simulink model "sampleModel1"  (R2021a)
settings: Solver=VariableStepAuto  StartTime=0.0  StopTime=50  RelTol=1e-3
undefined symbols (not defined in the file): DiscIntNeverNeededParam, magnitude, Newton, Raphson
libraries: simulink x92, pid_lib x10
(part 1 of 5)
settings Model: SimulationMode=accelerator  Creator=user  LastModifiedBy=O1

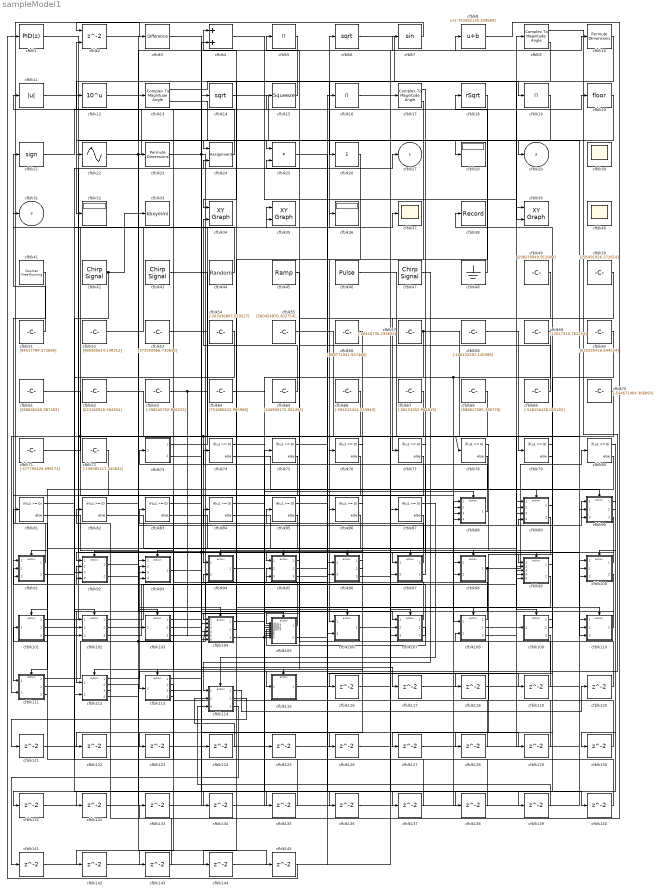
== system sampleModel1 ==
  cfblk1 : pid_lib/PID Controller  Controller=PID  Form=Parallel  TimeDomain=Discrete-time  UseExternalTs=off  SampleTime=1  IntegratorMethod=Forward Euler  FilterMethod=Forward Euler  ControllerParametersSource=internal  P=1  I=1  D=0  UseFilter=on  N=100  TunerSelectOption=Transfer Function Based (PID Tuner App)  InitialConditionSource=internal  InitialConditionForIntegrator=0  InitialConditionForFilter=0  DifferentiatorICPrevScaledInput=0  ExternalReset=none  TrackingMode=off  Kt=1  LimitOutput=off  SatLimitsSource=internal  UpperSaturationLimit=inf  LowerSaturationLimit=-inf  LinearizeAsGain=off  AntiWindupMode=none  Kb=1  POutMin=[]  POutMax=[]  IOutMin=[]  IOutMax=[]  DOutMin=[]  DOutMax=[]  NOutMin=[]  NOutMax=[]  SumOutMin=[]  SumOutMax=[]  SaturationOutMin=[]  SaturationOutMax=[]  PParamMin=[]  PParamMax=[]  IParamMin=[]  IParamMax=[]  DParamMin=[]  DParamMax=[]  NParamMin=[]  NParamMax=[]  KbParamMin=[]  KbParamMax=[]  KtParamMin=[]  KtParamMax=[]  KbOutMin=[]  KbOutMax=[]  KtOutMin=[]  KtOutMax=[]  IntegratorOutMin=[]  IntegratorOutMax=[]  FilterOutMin=[]  FilterOutMax=[]  SumI1OutMin=[]  SumI1OutMax=[]  SumI2OutMin=[]  SumI2OutMax=[]  SumI3OutMin=[]  SumI3OutMax=[]  SumI4OutMin=[]  SumI4OutMax=[]  SumDOutMin=[]  SumDOutMax=[]  DifferentiatorOutMin=[]  DifferentiatorOutMax=[]  FilterDiffOutCoefMin=[]  FilterDiffOutCoefMax=[]  ReciprocalOutMin=[]  ReciprocalOutMax=[]  SumDenOutMin=[]  SumDenOutMax=[]  SumNumOutMin=[]  SumNumOutMax=[]  DivideOutMin=[]  DivideOutMax=[]  UdiffTsProdOutMin=[]  UdiffTsProdOutMax=[]  NTsProdOutMin=[]  NTsProdOutMax=[]  UintegralTsProdOutMin=[]  UintegralTsProdOutMax=[]  UngainTsProdOutMin=[]  UngainTsProdOutMax=[]  IntegratorContinuousStateAttributes=''  IntegratorStateMustResolveToSignalObject=off  IntegratorRTWStateStorageClass=Auto  FilterContinuousStateAttributes=''  FilterStateMustResolveToSignalObject=off  FilterRTWStateStorageClass=Auto  ParallelPVariant=InternalParameters  IdealPVariant=Disabled  IVariant=InternalParameters  DVariant=InternalParameters  IntegratorVariant=Discrete  SatVariant=Disabled  AWVariant=Passthrough  PCopyVariant=Disabled  TRVariant=Disabled  FdbkBlocksVariant=Forward  IdealPFdbkVariant=Disabled  SatFdbkVariant=Disabled  DerivativeFilterVariant=ForwardEulerFilter  NVariant=InternalParameters  NCopyVariant=Disabled  FilterICVariant=InternalICsFilter  IntegratorICVariant=InternalICs  ExternalResetVariant=Disabled  TRSumVariant=Passthrough  SumFdbkVariant=Disabled  SumVariant=Sum_PID  TsampFilterVariant=InternalTs  TsampNgainVariant=Passthrough  TsampIntegralVariant=Passthrough  ExternalSaturationOutDataTypeStr=Inherit: Same as second input
  cfblk10 : PermuteDimensions
  cfblk100 : Subsystem  TreatAsAtomicUnit=on
  cfblk101 : Subsystem  TreatAsAtomicUnit=on
  cfblk102 : Subsystem  TreatAsAtomicUnit=on
  cfblk103 : Subsystem  TreatAsAtomicUnit=on
  cfblk104 : Subsystem  TreatAsAtomicUnit=on
  cfblk105 : Subsystem  TreatAsAtomicUnit=on
  cfblk106 : Subsystem  TreatAsAtomicUnit=on
  cfblk107 : Subsystem  TreatAsAtomicUnit=on
  cfblk108 : Subsystem  TreatAsAtomicUnit=on
  cfblk109 : Subsystem  TreatAsAtomicUnit=on
  cfblk11 : Abs
  cfblk110 : Subsystem  TreatAsAtomicUnit=on
  cfblk111 : Subsystem  TreatAsAtomicUnit=on
  cfblk112 : Subsystem  TreatAsAtomicUnit=on
  cfblk113 : Subsystem  TreatAsAtomicUnit=on
  cfblk114 : Subsystem  TreatAsAtomicUnit=on
  cfblk115 : Subsystem  TreatAsAtomicUnit=on
  cfblk{116..145} (30 alike) : Delay  SampleTime=1
  cfblk12 : Math  Operator=10^u  SaturateOnIntegerOverflow=on
  cfblk13 : ComplexToMagnitudeAngle
  cfblk14 : Sqrt  SaturateOnIntegerOverflow=on
  cfblk15 : Squeeze
  cfblk16 : Product  Inputs=*
  cfblk17 : ComplexToMagnitudeAngle
  cfblk18 : Sqrt  Operator=rSqrt  AlgorithmType=Newton-Raphson  SaturateOnIntegerOverflow=on
  cfblk19 : Product  Inputs=*
  cfblk2 : Delay  ShowEnablePort=on  SampleTime=1
      settings: InputPortMap=u0,e6
  cfblk20 : Rounding
  cfblk21 : Signum
  cfblk22 : Sin  TimeSource=Use external signal  SampleTime=0
  cfblk23 : PermuteDimensions
  cfblk24 : Assignment  DiagnosticForDimensions=Warning  IndexOptions=Index vector (dialog)  Indices=1  OutputSizes=1
  cfblk25 : DotProduct  InputSameDT=on  OutDataTypeStr=Inherit: Inherit via internal rule
  cfblk26 : Sum  Inputs=+
  cfblk28 : Display
  cfblk3 : simulink/Discrete/Difference  ICPrevInput=0.0  OutMin=[]  OutMax=[]  OutDataTypeStr=Inherit: Inherit via back propagation  OutDataType=fixdt(1, 16)  OutScaling=2^-10  DoSatur=off
  cfblk30 : Scope
      settings: Floating=on
  cfblk32 : Display
  cfblk33 : ToWorkspace  VariableName=kbxymmi  SaveFormat=Timeseries  SampleTime=-1
  cfblk34 : simulink/Sinks/XY Graph  xmin=-1  xmax=1  ymin=-1  ymax=1  st=-1
  cfblk35 : simulink/Sinks/XY Graph  xmin=-1  xmax=1  ymin=-1  ymax=1  st=-1
  cfblk36 : Display
  cfblk37 : Scope
  cfblk38 : Record  FileSettingsInternal="{\"entries\":[{\"content\":{\"excelSettings\":{\"content\":{},\"type\":\"Streamout.ExcelSettings\"}},\"type\":\"Streamout.FileSettingStorage\",\"uuid\":\"176fac1a-9541-496c-8a8b-0fabc606d681\"}],\"packageUris\":[\"http://schema.mathworks.com/mf0/streamout_blocks/R2020a\"],\"version\":\"1.0\"}"  SignalsInternal="{\"entries\":[{\"content\":{\"signals\":[{\"content\":{\"blockPath\":[\"sampleModel1/cfblk38\"],\"channel\":[],\"dimensions\":[1],\"domain\":\"samplemodel1/cfblk38\",\"lineColor\":\"#ff6929\",\"plots\":[1],\"port\":1,\"sid\":[],\"signalID\":15,\"signalName\":\"cfblk109:2\"},\"type\":\"RecordBlkView.Signal\",\"uuid\":\"c7513c56-5db2-4e4b-af3b-43bbc007c584\"}]},\"type\":\"RecordBlkView.InputSignals\",\"uuid\":\"33f00b58-3736-4c4e-bce4-d943bd5669e6\"}],\"packageUris\":[\"http://schema.mathworks.com/mf0/streamout_blocks/R2020a\"],\"version\":\"1.0\"}"  VisualizationBindings="{\"sparklinesplugin\":{\"info\":[{\"bindingParametersList\":[],\"subplotID\":1}]}}"
  cfblk39 : simulink/Sinks/XY Graph  xmin=-1  xmax=1  ymin=-1  ymax=1  st=-1
  cfblk4 : Sum
  cfblk40 : Scope
      settings: Floating=on
  cfblk41 : simulink/Sources/Counter Free-Running  NumBits=[54.000000]  tsamp=-1
  cfblk42 : simulink/Sources/Chirp Signal  f1=[-261506437.759570]  T=[-777594489.412425]  f2=[560504136.642276]
  cfblk43 : simulink/Sources/Chirp Signal  f1=[-220522326.077493]  T=[-516617428.172335]  f2=[-192175708.823771]
  cfblk44 : RandomNumber  Mean=[-80709.094966]  Variance=[13197.329261]  Seed=[942050590.000000]  SampleTime=0.1
  cfblk45 : simulink/Sources/Ramp  slope=[9122.690805]  start=[29.185221]  InitialOutput=[-880440.914106]
  cfblk46 : DiscretePulseGenerator  PulseType=Time based  Amplitude=[-530440173.255187]  Period=[35315857.769049]  PulseWidth=5  PhaseDelay=[8.000000]
  cfblk47 : simulink/Sources/Chirp Signal  f1=[-969193124.696890]  T=[-913952396.684384]  f2=[-662019941.074591]
  cfblk48 : Ground
  cfblk49 : Constant  Value=[298230949.912904]  SampleTime=1
  cfblk5 : Product  Inputs=*
  cfblk50 : Constant  Value=[295491926.272614]  SampleTime=1
  cfblk51 : Constant  Value=[94017784.572690]  SampleTime=1
  cfblk52 : Constant  Value=[489385614.148312]  SampleTime=1
  cfblk53 : Constant  Value=[373550866.730630]  SampleTime=1
  cfblk54 : Constant  Value=[-263030807.019327]  SampleTime=1
  cfblk55 : Constant  Value=[560454870.302754]  SampleTime=1
  cfblk56 : Constant  Value=[858771941.937460]  SampleTime=1
  cfblk57 : Constant  Value=[-26416735.193655]  SampleTime=1
  cfblk58 : Constant  Value=[-106432501.140388]  SampleTime=1
  cfblk59 : Constant  Value=[17017310.762254]  SampleTime=1
  cfblk6 : Sqrt  SaturateOnIntegerOverflow=on
  cfblk60 : Constant  Value=[635255416.644524]  SampleTime=1
  cfblk61 : Constant  Value=[288636260.387383]  SampleTime=1
  cfblk62 : Constant  Value=[623160916.564954]  SampleTime=1
  cfblk63 : Constant  Value=[-298545792.846233]  SampleTime=1
  cfblk64 : Constant  Value=[751885622.985968]  SampleTime=1
  cfblk65 : Constant  Value=[244950172.002455]  SampleTime=1
  cfblk66 : Constant  Value=[-584515414.533943]  SampleTime=1
  cfblk67 : Constant  Value=[-58153302.964819]  SampleTime=1
  cfblk68 : Constant  Value=[688617585.390778]  SampleTime=1
  cfblk69 : Constant  Value=[-548156438.055202]  SampleTime=1
  cfblk7 : Trigonometry
  cfblk70 : Constant  Value=[-544671404.366893]  SampleTime=1
  cfblk71 : Constant  Value=[-377795426.699174]  SampleTime=1
  cfblk72 : Constant  Value=[-139585217.340832]  SampleTime=1
  cfblk73 : Subsystem
  cfblk{74..87} (14 alike) : If  IfExpression=u1 >= 0  SampleTime=1
  cfblk8 : Bias  Bias=[-753362130.329669]
  cfblk88 : Subsystem  TreatAsAtomicUnit=on
  cfblk89 : Subsystem  TreatAsAtomicUnit=on
  cfblk9 : ComplexToMagnitudeAngle
  cfblk90 : Subsystem  TreatAsAtomicUnit=on
  cfblk91 : Subsystem  TreatAsAtomicUnit=on
  cfblk92 : Subsystem  TreatAsAtomicUnit=on
  cfblk93 : Subsystem  TreatAsAtomicUnit=on
  cfblk94 : Subsystem  TreatAsAtomicUnit=on
  cfblk95 : Subsystem  TreatAsAtomicUnit=on
  cfblk96 : Subsystem  TreatAsAtomicUnit=on
  cfblk97 : Subsystem  TreatAsAtomicUnit=on
  cfblk98 : Subsystem  TreatAsAtomicUnit=on
  cfblk99 : Subsystem  TreatAsAtomicUnit=on
  cfblk27 : Outport
  cfblk29 : Outport  Port=2
  cfblk31 : Outport  Port=3
  wires:
  cfblk42/1 -> cfblk33/1, cfblk102/3(cfblk10)
  cfblk98/1(cfblk2) -> cfblk80/1, cfblk104/6(cfblk15)
  cfblk1/1 -> cfblk100/2(cfblk8)
  cfblk91/1(cfblk2) -> cfblk3/1
  cfblk61/1 -> cfblk78/1, cfblk99/3(cfblk12)
  cfblk13/1 -> cfblk19/1
  cfblk9/1 -> cfblk115/1(cfblk1)
  cfblk73/1(cfblk2) -> cfblk6/1
  cfblk14/1 -> cfblk28/1
  cfblk52/1 -> cfblk37/1
  cfblk97/1(cfblk2) -> cfblk85/1
  cfblk13/2 -> cfblk110/1(cfblk1)
  cfblk51/1 -> cfblk21/1
  cfblk47/1 -> cfblk114/1(cfblk1)
  cfblk23/1 -> cfblk99/4(cfblk13), cfblk105/7(cfblk12), cfblk107/1(cfblk1)
  cfblk115/1(cfblk2) -> cfblk17/1
  cfblk72/1 -> cfblk111/1(cfblk1)
  cfblk49/1 -> cfblk77/1
  cfblk100/1(cfblk2) -> cfblk97/1(cfblk1)
  cfblk7/1 -> cfblk2/1
  cfblk101/1(cfblk2) -> cfblk27/1
  cfblk71/1 -> cfblk13/1
  cfblk10/1 -> cfblk26/1
  cfblk68/1 -> cfblk106/1(cfblk1)
  cfblk19/1 -> cfblk25/1
  cfblk9/2 -> cfblk32/1
  cfblk41/1 -> cfblk91/1(cfblk1)
  cfblk46/1 -> cfblk98/1(cfblk1)
  cfblk6/1 -> cfblk39/1
  cfblk24/1 -> cfblk2/2
  cfblk11/1 -> cfblk24/1
  cfblk5/1 -> cfblk34/1
  cfblk16/1 -> cfblk10/1
  cfblk55/1 -> cfblk108/1(cfblk1)
  cfblk59/1 -> cfblk88/2(cfblk8), cfblk105/6(cfblk11)
  cfblk100/2(cfblk10) -> cfblk112/1(cfblk1)
  cfblk62/1 -> cfblk94/1(cfblk1), cfblk99/5(cfblk14)
  cfblk20/1 -> cfblk22/1
  cfblk111/1(cfblk2) -> cfblk16/1
  cfblk108/1(cfblk2) -> cfblk4/1
  cfblk105/1(cfblk2) -> cfblk84/1
  cfblk58/1 -> cfblk79/1
  cfblk60/1 -> cfblk99/1(cfblk1)
  cfblk45/1 -> cfblk105/1(cfblk1)
  cfblk102/1(cfblk2) -> cfblk14/1
  cfblk70/1 -> cfblk107/3(cfblk14)
  cfblk108/2(cfblk11) -> cfblk89/2(cfblk12)
  cfblk73/2(cfblk16) -> cfblk36/1
  cfblk88/1(cfblk2) -> cfblk25/2
  cfblk12/1 -> cfblk7/1
  cfblk95/1(cfblk2) -> cfblk94/2(cfblk8)
  cfblk93/1(cfblk2) -> cfblk8/1
  cfblk108/3(cfblk12) -> cfblk89/3(cfblk13)
  cfblk50/1 -> cfblk95/1(cfblk1)
  cfblk15/1 -> cfblk12/1
  cfblk65/1 -> cfblk34/2
  cfblk18/1 -> cfblk76/1
  cfblk22/1 -> cfblk9/1, cfblk104/4(cfblk13)
  cfblk53/1 -> cfblk98/2(cfblk7)
  cfblk2/1 -> cfblk29/1
  cfblk104/2(cfblk16) -> cfblk91/2(cfblk13)
  cfblk67/1 -> cfblk105/2(cfblk7)
  cfblk48/1 -> cfblk18/1
  cfblk69/1 -> cfblk5/1
  cfblk105/2(cfblk14) -> cfblk89/4(cfblk14)
  cfblk92/1(cfblk2) -> cfblk23/1
  cfblk107/1(cfblk2) -> cfblk11/1
  cfblk56/1 -> cfblk86/1
  cfblk21/1 -> cfblk15/1
  cfblk54/1 -> cfblk112/2(cfblk7)
  cfblk89/2(cfblk15) -> cfblk113/1(cfblk1)
  cfblk66/1 -> cfblk111/2(cfblk13)
  cfblk102/2(cfblk11) -> cfblk4/2
  cfblk112/1(cfblk2) -> cfblk93/2(cfblk14)
  cfblk109/2(cfblk11) -> cfblk38/1
  cfblk104/3(cfblk17) -> cfblk90/3(cfblk12), cfblk129/1
  cfblk4/1 -> cfblk39/2
  cfblk97/2(cfblk11) -> cfblk73/1(cfblk1)
  cfblk111/2(cfblk14) -> cfblk24/2
  cfblk17/1 -> cfblk92/1(cfblk1)
  cfblk102/3(cfblk12) -> cfblk20/1
  cfblk63/1 -> cfblk110/3(cfblk8), cfblk104/5(cfblk14)
  cfblk113/3(cfblk12) -> cfblk95/2(cfblk9)
  cfblk111/3(cfblk15) -> cfblk81/1
  cfblk91/2(cfblk15) -> cfblk35/1
  cfblk107/2(cfblk15) -> cfblk105/4(cfblk9)
  cfblk103/3(cfblk7) -> cfblk95/3(cfblk10)
  cfblk44/1 -> cfblk31/1
  cfblk101/3(cfblk14) -> cfblk35/2
  cfblk107/3(cfblk16) -> cfblk91/3(cfblk14)
  cfblk110/1(cfblk2) -> cfblk102/2(cfblk9)
  cfblk26/1 -> cfblk104/1(cfblk1)
  cfblk112/3(cfblk9) -> cfblk92/2(cfblk13)
  cfblk43/1 -> cfblk106/2(cfblk7)
  cfblk112/4(cfblk10) -> cfblk90/1(cfblk1), cfblk104/3(cfblk12)
  cfblk57/1 -> cfblk90/2(cfblk11), cfblk105/8(cfblk13)
  cfblk92/2(cfblk16) -> cfblk93/3(cfblk15)
  cfblk64/1 -> cfblk105/5(cfblk10)
  cfblk90/3(cfblk14) -> cfblk99/2(cfblk11)
  cfblk74/1 -> cfblk88/Action
  cfblk74/2 -> cfblk89/Action
  cfblk75/1 -> cfblk90/Action
  cfblk75/2 -> cfblk91/Action
  cfblk76/1 -> cfblk92/Action
  cfblk76/2 -> cfblk93/Action
  cfblk77/1 -> cfblk94/Action
  cfblk77/2 -> cfblk95/Action
  cfblk78/1 -> cfblk96/Action
  cfblk78/2 -> cfblk97/Action
  cfblk79/1 -> cfblk98/Action
  cfblk79/2 -> cfblk99/Action
  cfblk80/1 -> cfblk100/Action
  cfblk80/2 -> cfblk101/Action
  cfblk81/1 -> cfblk102/Action
  cfblk81/2 -> cfblk103/Action
  cfblk82/1 -> cfblk104/Action
  cfblk82/2 -> cfblk105/Action
  cfblk83/1 -> cfblk106/Action
  cfblk83/2 -> cfblk107/Action
  cfblk84/1 -> cfblk108/Action
  cfblk84/2 -> cfblk109/Action
  cfblk85/1 -> cfblk110/Action
  cfblk85/2 -> cfblk111/Action
  cfblk86/1 -> cfblk112/Action
  cfblk86/2 -> cfblk113/Action
  cfblk87/1 -> cfblk114/Action
  cfblk87/2 -> cfblk115/Action
  cfblk89/1(cfblk2) -> cfblk116/1
  cfblk116/1 -> cfblk107/2(cfblk13)
  cfblk113/1(cfblk2) -> cfblk117/1
  cfblk117/1 -> cfblk89/1(cfblk1)
  cfblk25/1 -> cfblk118/1
  cfblk118/1 -> cfblk100/3(cfblk9)
  cfblk106/1(cfblk2) -> cfblk119/1
  cfblk119/1 -> cfblk74/1
  cfblk114/1(cfblk2) -> cfblk120/1
  cfblk120/1 -> cfblk83/1
  cfblk114/2(cfblk14) -> cfblk121/1
  cfblk121/1 -> cfblk96/1(cfblk1)
  cfblk96/1(cfblk2) -> cfblk122/1
  cfblk122/1 -> cfblk88/4(cfblk10)
  cfblk96/2(cfblk13) -> cfblk123/1
  cfblk123/1 -> cfblk103/1(cfblk1)
  cfblk103/1(cfblk2) -> cfblk124/1
  cfblk124/1 -> cfblk114/2(cfblk12)
  cfblk104/1(cfblk2) -> cfblk125/1
  cfblk125/1 -> cfblk100/1(cfblk1)
  cfblk3/1 -> cfblk126/1
  cfblk126/1 -> cfblk109/1(cfblk1)
  cfblk109/1(cfblk2) -> cfblk127/1
  cfblk127/1 -> cfblk88/3(cfblk9)
  cfblk109/3(cfblk12) -> cfblk128/1
  cfblk128/1 -> cfblk92/3(cfblk14)
  cfblk129/1 -> cfblk105/3(cfblk8)
  cfblk90/1(cfblk2) -> cfblk130/1
  cfblk130/1 -> cfblk108/2(cfblk10)
  cfblk90/2(cfblk13) -> cfblk131/1
  cfblk131/1 -> cfblk104/2(cfblk11)
  cfblk99/1(cfblk2) -> cfblk132/1
  cfblk132/1 -> cfblk93/1(cfblk1)
  cfblk8/1 -> cfblk133/1
  cfblk133/1 -> cfblk75/1
  cfblk99/2(cfblk15) -> cfblk134/1
  cfblk134/1 -> cfblk110/2(cfblk7)
  cfblk103/2(cfblk6) -> cfblk135/1
  cfblk135/1 -> cfblk82/1
  cfblk94/1(cfblk2) -> cfblk136/1
  cfblk136/1 -> cfblk88/1(cfblk1)
  cfblk95/2(cfblk11) -> cfblk137/1
  cfblk137/1 -> cfblk101/1(cfblk1)
  cfblk101/2(cfblk13) -> cfblk138/1
  cfblk138/1 -> cfblk102/1(cfblk1)
  cfblk95/3(cfblk12) -> cfblk139/1
  cfblk139/1 -> cfblk114/3(cfblk13)
  cfblk96/3(cfblk14) -> cfblk140/1
  cfblk140/1 -> cfblk93/4(cfblk16)
  cfblk114/3(cfblk15) -> cfblk141/1
  cfblk141/1 -> cfblk96/2(cfblk12)
  cfblk113/2(cfblk11) -> cfblk142/1
  cfblk142/1 -> cfblk87/1
  cfblk113/4(cfblk13) -> cfblk143/1
  cfblk143/1 -> cfblk92/4(cfblk15)
  cfblk17/2 -> cfblk144/1
  cfblk144/1 -> cfblk97/2(cfblk10)
  cfblk112/2(cfblk8) -> cfblk145/1
  cfblk145/1 -> cfblk1/1

== system sampleModel1/cfblk100 ==
  cfblk1 : Inport
  cfblk8 : Inport  Port=2
  cfblk9 : Inport  Port=3
  Action Port : ActionPort  ActionPortLabel=if(u1 >= 0)
  cfblk3 : simulink/Discrete/Transfer Fcn Lead or Lag  PoleZ=0.95  ZeroZ=0.75  ICPrevOutput=0.0  ICPrevInput=0.0  DoSatur=off
      settings: SourceProductBaseCode=SL
  cfblk4 : Reshape
  cfblk5 : Signum
  cfblk6 : Rounding
  cfblk7 : Constant  Value=[458643452.487135]  SampleTime=1
  cfblk2 : Outport
  cfblk10 : Outport  Port=2
  wires:
  cfblk3/1 -> cfblk5/1
  cfblk1/1 -> cfblk4/1
  cfblk4/1 -> cfblk10/1
  cfblk7/1 -> cfblk3/1
  cfblk9/1 -> cfblk2/1
  cfblk5/1 -> cfblk6/1

== system sampleModel1/cfblk101 ==
  cfblk1 : Inport
  Action Port : ActionPort  ActionPortLabel=else
  cfblk10 : Trigonometry
  cfblk11 : Constant  Value=[951414251.341264]  SampleTime=1
  cfblk12 : Subsystem
  cfblk15 : Delay
  cfblk16 : Delay
  cfblk3 : Delay  DelayLengthSource=Input port
      settings: InputPortMap=u0,p1
  cfblk4 : DiscreteFir
  cfblk5 : Product
  cfblk6 : Sum  Inputs=|++
  cfblk7 : Sum  Inputs=+
  cfblk8 : ComplexToRealImag
  cfblk9 : Rounding
  cfblk2 : Outport
  cfblk13 : Outport  Port=2
  cfblk14 : Outport  Port=3
  wires:
  cfblk11/1 -> cfblk4/1, cfblk6/2, cfblk14/1
  cfblk5/1 -> cfblk7/1
  cfblk10/1 -> cfblk3/2, cfblk15/1
  cfblk9/1 -> cfblk12/2(cfblk6)
  cfblk4/1 -> cfblk3/1, cfblk8/1
  cfblk12/1(cfblk2) -> cfblk10/1
  cfblk3/1 -> cfblk13/1
  cfblk1/1 -> cfblk2/1
  cfblk12/2(cfblk8) -> cfblk6/1
  cfblk8/1 -> cfblk5/2
  cfblk7/1 -> cfblk9/1
  cfblk8/2 -> cfblk12/3(cfblk7)
  cfblk15/1 -> cfblk5/1
  cfblk6/1 -> cfblk16/1
  cfblk16/1 -> cfblk12/1(cfblk1)

== system sampleModel1/cfblk102 ==
  cfblk1 : Inport
  cfblk9 : Inport  Port=2
  cfblk10 : Inport  Port=3
  Action Port : ActionPort  ActionPortLabel=if(u1 >= 0)
  cfblk3 : Constant  Value=[-893999894.979913]  SampleTime=1
  cfblk4 : Constant  Value=[595971915.355237]  SampleTime=1
  cfblk5 : Constant  Value=[-935328893.107163]  SampleTime=1
  cfblk6 : Constant  Value=[439603109.784381]  SampleTime=1
  cfblk7 : Constant  Value=[-566705247.439443]  SampleTime=1
  cfblk8 : Constant  Value=[-722676234.261465]  SampleTime=1
  cfblk2 : Outport
  cfblk11 : Outport  Port=2
  cfblk12 : Outport  Port=3
  wires:
  cfblk1/1 -> cfblk12/1
  cfblk4/1 -> cfblk2/1
  cfblk3/1 -> cfblk11/1

== system sampleModel1/cfblk103 ==
  cfblk1 : Inport
  Action Port : ActionPort  ActionPortLabel=else
  cfblk3 : Product  Inputs=**
  cfblk4 : Sum  Inputs=-+
  cfblk5 : Subsystem
  cfblk8 : Delay
  cfblk9 : Delay
  cfblk2 : Outport
  cfblk6 : Outport  Port=2
  cfblk7 : Outport  Port=3
  wires:
  cfblk1/1 -> cfblk6/1
  cfblk5/1(cfblk2) -> cfblk4/1
  cfblk5/2(cfblk15) -> cfblk4/2
  cfblk3/1 -> cfblk7/1, cfblk5/1(cfblk1), cfblk5/2(cfblk12), cfblk5/3(cfblk13), cfblk5/4(cfblk14)
  cfblk5/4(cfblk17) -> cfblk2/1
  cfblk4/1 -> cfblk8/1
  cfblk8/1 -> cfblk3/1
  cfblk5/3(cfblk16) -> cfblk9/1
  cfblk9/1 -> cfblk3/2

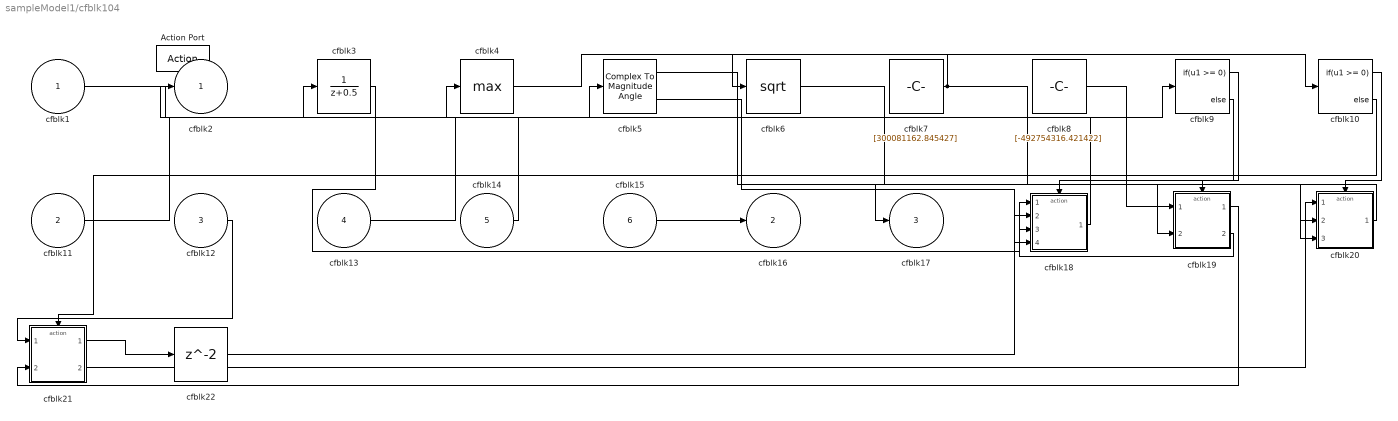
== system sampleModel1/cfblk104 ==
  cfblk1 : Inport
  cfblk11 : Inport  Port=2
  cfblk12 : Inport  Port=3
  cfblk13 : Inport  Port=4
  cfblk14 : Inport  Port=5
  cfblk15 : Inport  Port=6
  Action Port : ActionPort  ActionPortLabel=if(u1 >= 0)
  cfblk10 : If  IfExpression=u1 >= 0  SampleTime=1
  cfblk18 : Subsystem  TreatAsAtomicUnit=on
  cfblk19 : Subsystem  TreatAsAtomicUnit=on
  cfblk20 : Subsystem  TreatAsAtomicUnit=on
  cfblk21 : Subsystem  TreatAsAtomicUnit=on
  cfblk22 : Delay
  cfblk3 : DiscreteTransferFcn
  cfblk4 : MinMax  Function=max
  cfblk5 : ComplexToMagnitudeAngle
  cfblk6 : Sqrt  SaturateOnIntegerOverflow=on
  cfblk7 : Constant  Value=[300081162.845427]  SampleTime=1
  cfblk8 : Constant  Value=[-492754316.421422]  SampleTime=1
  cfblk9 : If  IfExpression=u1 >= 0  SampleTime=1
  cfblk2 : Outport
  cfblk16 : Outport  Port=2
  cfblk17 : Outport  Port=3
  wires:
  cfblk13/1 -> cfblk5/1
  cfblk4/1 -> cfblk10/1
  cfblk18/1(cfblk2) -> cfblk4/1
  cfblk3/1 -> cfblk18/1(cfblk1)
  cfblk8/1 -> cfblk19/1(cfblk1)
  cfblk15/1 -> cfblk16/1
  cfblk1/1 -> cfblk9/1
  cfblk14/1 -> cfblk2/1
  cfblk11/1 -> cfblk3/1
  cfblk5/1 -> cfblk19/2(cfblk15)
  cfblk12/1 -> cfblk21/1(cfblk1)
  cfblk19/1(cfblk2) -> cfblk21/2(cfblk9)
  cfblk7/1 -> cfblk6/1, cfblk20/3(cfblk12)
  cfblk20/1(cfblk2) -> cfblk17/1
  cfblk19/2(cfblk16) -> cfblk18/3(cfblk7)
  cfblk5/2 -> cfblk18/4(cfblk8)
  cfblk21/2(cfblk10) -> cfblk20/1(cfblk1)
  cfblk6/1 -> cfblk20/2(cfblk11)
  cfblk9/1 -> cfblk18/Action
  cfblk9/2 -> cfblk19/Action
  cfblk10/1 -> cfblk20/Action
  cfblk10/2 -> cfblk21/Action
  cfblk21/1(cfblk2) -> cfblk22/1
  cfblk22/1 -> cfblk18/2(cfblk6)

== system sampleModel1/cfblk105 ==
  cfblk1 : Inport
  cfblk7 : Inport  Port=2
  cfblk8 : Inport  Port=3
  cfblk9 : Inport  Port=4
  cfblk10 : Inport  Port=5
  cfblk11 : Inport  Port=6
  cfblk12 : Inport  Port=7
  cfblk13 : Inport  Port=8
  Action Port : ActionPort  ActionPortLabel=else
  cfblk3 : Rounding
  cfblk4 : Sum  Inputs=|++
  cfblk5 : simulink/Math Operations/Slider Gain  gain=1  low=0  high=2
  cfblk6 : Subsystem
  cfblk2 : Outport
  cfblk14 : Outport  Port=2
  wires:
  cfblk13/1 -> cfblk3/1
  cfblk10/1 -> cfblk5/1
  cfblk4/1 -> cfblk6/1(cfblk1)
  cfblk9/1 -> cfblk4/1
  cfblk12/1 -> cfblk14/1
  cfblk1/1 -> cfblk2/1
  cfblk7/1 -> cfblk4/2

== system sampleModel1/cfblk106 ==
  cfblk1 : Inport
  cfblk7 : Inport  Port=2
  Action Port : ActionPort  ActionPortLabel=if(u1 >= 0)
  cfblk3 : Product  Inputs=**
  cfblk4 : Sqrt  Operator=rSqrt  AlgorithmType=Newton-Raphson  SaturateOnIntegerOverflow=on
  cfblk5 : Constant  Value=[-792057482.954499]  SampleTime=1
  cfblk6 : Constant  Value=[297180528.830524]  SampleTime=1
  cfblk2 : Outport
  wires:
  cfblk1/1 -> cfblk4/1
  cfblk4/1 -> cfblk3/1
  cfblk6/1 -> cfblk2/1
  cfblk7/1 -> cfblk3/2

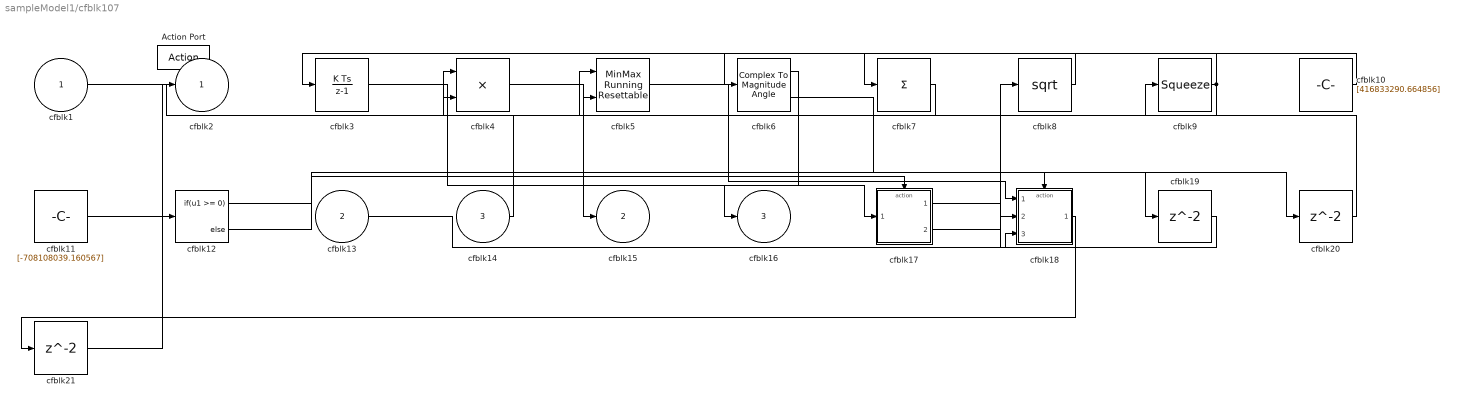
== system sampleModel1/cfblk107 ==
  cfblk1 : Inport
  cfblk13 : Inport  Port=2
  cfblk14 : Inport  Port=3
  Action Port : ActionPort  ActionPortLabel=else
  cfblk10 : Constant  Value=[416833290.664856]  SampleTime=1
  cfblk11 : Constant  Value=[-708108039.160567]  SampleTime=1
  cfblk12 : If  IfExpression=u1 >= 0  SampleTime=1
  cfblk17 : Subsystem  TreatAsAtomicUnit=on
  cfblk18 : Subsystem  TreatAsAtomicUnit=on
  cfblk19 : Delay
  cfblk20 : Delay
  cfblk21 : Delay
  cfblk3 : DiscreteIntegrator  SampleTime=-1  ICPrevOutput=DiscIntNeverNeededParam  ICPrevScaledInput=DiscIntNeverNeededParam
  cfblk4 : Product  Inputs=**
  cfblk5 : simulink/Math Operations/MinMax Running Resettable  Function=min  vinit=0.0
  cfblk6 : ComplexToMagnitudeAngle
  cfblk7 : Sum  Inputs=+
  cfblk8 : Sqrt  SaturateOnIntegerOverflow=on
  cfblk9 : Squeeze
  cfblk2 : Outport
  cfblk15 : Outport  Port=2
  cfblk16 : Outport  Port=3
  wires:
  cfblk10/1 -> cfblk3/1
  cfblk1/1 -> cfblk9/1
  cfblk5/1 -> cfblk18/1(cfblk1)
  cfblk8/1 -> cfblk6/1
  cfblk11/1 -> cfblk2/1
  cfblk9/1 -> cfblk7/1, cfblk5/2
  cfblk14/1 -> cfblk4/1
  cfblk17/2(cfblk8) -> cfblk8/1
  cfblk4/1 -> cfblk15/1
  cfblk3/1 -> cfblk17/1(cfblk1)
  cfblk7/1 -> cfblk4/2
  cfblk13/1 -> cfblk18/3(cfblk7)
  cfblk6/1 -> cfblk16/1
  cfblk12/1 -> cfblk17/Action
  cfblk12/2 -> cfblk18/Action
  cfblk17/1(cfblk2) -> cfblk19/1
  cfblk19/1 -> cfblk18/2(cfblk6)
  cfblk6/2 -> cfblk20/1
  cfblk20/1 -> cfblk5/1
  cfblk18/1(cfblk2) -> cfblk21/1
  cfblk21/1 -> cfblk12/1

== system sampleModel1/cfblk108 ==
  cfblk1 : Inport
  cfblk10 : Inport  Port=2
  Action Port : ActionPort  ActionPortLabel=if(u1 >= 0)
  cfblk13 : Delay
  cfblk3 : Assignment  DiagnosticForDimensions=Warning  IndexOptions=Index vector (dialog)  Indices=1  OutputSizes=1
  cfblk4 : Product  Inputs=*
  cfblk5 : simulink/Math Operations/MinMax Running Resettable  Function=min  vinit=0.0
  cfblk6 : Constant  Value=[234306988.918071]  SampleTime=1
  cfblk7 : Constant  Value=[-548298623.600525]  SampleTime=1
  cfblk8 : Constant  Value=[-980044687.900619]  SampleTime=1
  cfblk9 : Subsystem
  cfblk2 : Outport
  cfblk11 : Outport  Port=2
  cfblk12 : Outport  Port=3
  wires:
  cfblk1/1 -> cfblk5/1
  cfblk6/1 -> cfblk5/2
  cfblk8/1 -> cfblk4/1
  cfblk3/1 -> cfblk2/1, cfblk13/1
  cfblk7/1 -> cfblk9/1(cfblk1)
  cfblk4/1 -> cfblk11/1
  cfblk10/1 -> cfblk12/1
  cfblk9/1(cfblk2) -> cfblk3/1
  cfblk5/1 -> cfblk9/2(cfblk8)
  cfblk9/2(cfblk10) -> cfblk3/2
  cfblk13/1 -> cfblk9/3(cfblk9)

== system sampleModel1/cfblk109 ==
  cfblk1 : Inport
  Action Port : ActionPort  ActionPortLabel=else
  cfblk10 : Subsystem
  cfblk3 : PermuteDimensions
  cfblk4 : Reshape
  cfblk5 : Constant  Value=[69282507.073152]  SampleTime=1
  cfblk6 : Constant  Value=[746900198.161383]  SampleTime=1
  cfblk7 : Constant  Value=[-199940568.760723]  SampleTime=1
  cfblk8 : Constant  Value=[-876350571.175328]  SampleTime=1
  cfblk9 : Constant  Value=[-763028016.877942]  SampleTime=1
  cfblk2 : Outport
  cfblk11 : Outport  Port=2
  cfblk12 : Outport  Port=3
  wires:
  cfblk8/1 -> cfblk4/1
  cfblk1/1 -> cfblk2/1
  cfblk6/1 -> cfblk11/1
  cfblk7/1 -> cfblk10/1(cfblk1)
  cfblk10/1(cfblk2) -> cfblk12/1
  cfblk5/1 -> cfblk10/2(cfblk13)
  cfblk3/1 -> cfblk10/3(cfblk14)
  cfblk4/1 -> cfblk3/1
  cfblk9/1 -> cfblk10/4(cfblk15)

== system sampleModel1/cfblk110 ==
  cfblk1 : Inport
  cfblk7 : Inport  Port=2
  cfblk8 : Inport  Port=3
  Action Port : ActionPort  ActionPortLabel=if(u1 >= 0)
  cfblk3 : Rounding
  cfblk4 : Sum  Inputs=+
  cfblk5 : Constant  Value=[-878619225.133228]  SampleTime=1
  cfblk6 : Constant  Value=[-167336281.956525]  SampleTime=1
  cfblk2 : Outport
  wires:
  cfblk1/1 -> cfblk4/1
  cfblk5/1 -> cfblk2/1
  cfblk7/1 -> cfblk3/1

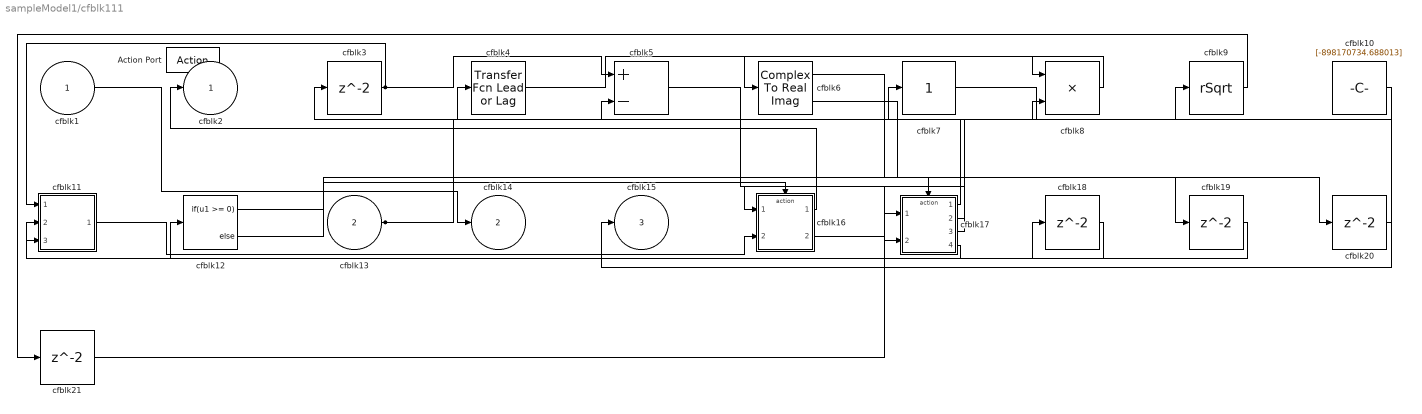
== system sampleModel1/cfblk111 ==
  cfblk1 : Inport
  cfblk13 : Inport  Port=2
  Action Port : ActionPort  ActionPortLabel=else
  cfblk10 : Constant  Value=[-898170734.688013]  SampleTime=1
  cfblk11 : Subsystem
  cfblk12 : If  IfExpression=u1 >= 0  SampleTime=1
  cfblk16 : Subsystem  TreatAsAtomicUnit=on
  cfblk17 : Subsystem  TreatAsAtomicUnit=on
  cfblk{3,18..21} (5 alike) : Delay
  cfblk4 : simulink/Discrete/Transfer Fcn Lead or Lag  PoleZ=0.95  ZeroZ=0.75  ICPrevOutput=0.0  ICPrevInput=0.0  DoSatur=off
      settings: SourceProductBaseCode=SL
  cfblk5 : Sum  Inputs=+-
  cfblk6 : ComplexToRealImag
  cfblk7 : simulink/Math Operations/Slider Gain  gain=1  low=0  high=2
  cfblk8 : Product
  cfblk9 : Sqrt  Operator=rSqrt  AlgorithmType=Newton-Raphson  SaturateOnIntegerOverflow=on
  cfblk2 : Outport
  cfblk14 : Outport  Port=2
  cfblk15 : Outport  Port=3
  wires:
  cfblk8/1 -> cfblk6/1
  cfblk17/1(cfblk2) -> cfblk4/1
  cfblk16/1(cfblk2) -> cfblk2/1
  cfblk1/1 -> cfblk14/1
  cfblk5/1 -> cfblk17/2(cfblk13)
  cfblk10/1 -> cfblk15/1
  cfblk7/1 -> cfblk9/1
  cfblk4/1 -> cfblk8/1
  cfblk3/1 -> cfblk11/1(cfblk1), cfblk5/1
  cfblk13/1 -> cfblk8/2, cfblk5/2
  cfblk17/2(cfblk14) -> cfblk7/1
  cfblk17/3(cfblk15) -> cfblk16/1(cfblk1)
  cfblk17/4(cfblk16) -> cfblk11/2(cfblk9)
  cfblk11/1(cfblk2) -> cfblk16/2(cfblk6)
  cfblk12/1 -> cfblk16/Action
  cfblk12/2 -> cfblk17/Action
  cfblk16/2(cfblk7) -> cfblk18/1
  cfblk18/1 -> cfblk11/3(cfblk10)
  cfblk6/1 -> cfblk19/1
  cfblk19/1 -> cfblk12/1
  cfblk6/2 -> cfblk20/1
  cfblk20/1 -> cfblk3/1
  cfblk9/1 -> cfblk21/1
  cfblk21/1 -> cfblk17/1(cfblk1)

== system sampleModel1/cfblk112 ==
  cfblk1 : Inport
  cfblk7 : Inport  Port=2
  Action Port : ActionPort  ActionPortLabel=if(u1 >= 0)
  cfblk11 : Subsystem  TreatAsAtomicUnit=on
  cfblk12 : Subsystem  TreatAsAtomicUnit=on
  cfblk13 : Delay
  cfblk3 : Bias  Bias=[261451486.736793]
  cfblk4 : Constant  Value=[-259791308.572268]  SampleTime=1
  cfblk5 : Constant  Value=[591388662.386798]  SampleTime=1
  cfblk6 : If  IfExpression=u1 >= 0  SampleTime=1
  cfblk2 : Outport
  cfblk8 : Outport  Port=2
  cfblk9 : Outport  Port=3
  cfblk10 : Outport  Port=4
  wires:
  cfblk12/1(cfblk2) -> cfblk11/1(cfblk1), cfblk8/1
  cfblk5/1 -> cfblk2/1
  cfblk4/1 -> cfblk11/2(cfblk12)
  cfblk1/1 -> cfblk9/1, cfblk12/3(cfblk10)
  cfblk7/1 -> cfblk3/1, cfblk12/2(cfblk9)
  cfblk3/1 -> cfblk10/1, cfblk12/1(cfblk1)
  cfblk6/1 -> cfblk11/Action
  cfblk6/2 -> cfblk12/Action
  cfblk11/1(cfblk2) -> cfblk13/1
  cfblk13/1 -> cfblk6/1

== system sampleModel1/cfblk113 ==
  cfblk1 : Inport
  Action Port : ActionPort  ActionPortLabel=else
  cfblk10 : Constant  Value=[-294378378.783245]  SampleTime=1
  cfblk3 : DiscreteIntegrator  SampleTime=-1  ICPrevOutput=DiscIntNeverNeededParam  ICPrevScaledInput=DiscIntNeverNeededParam
  cfblk4 : Trigonometry
  cfblk5 : Sum  Inputs=|++
  cfblk6 : Assignment  DiagnosticForDimensions=Warning  IndexOptions=Index vector (dialog)  Indices=1  OutputSizes=1
  cfblk7 : Squeeze
  cfblk8 : simulink/Math Operations/MinMax Running Resettable  Function=min  vinit=0.0
  cfblk9 : Constant  Value=[56024317.637537]  SampleTime=1
  cfblk2 : Outport
  cfblk11 : Outport  Port=2
  cfblk12 : Outport  Port=3
  cfblk13 : Outport  Port=4
  wires:
  cfblk10/1 -> cfblk7/1
  cfblk1/1 -> cfblk3/1
  cfblk7/1 -> cfblk6/1
  cfblk4/1 -> cfblk13/1, cfblk8/2
  cfblk9/1 -> cfblk6/2, cfblk12/1
  cfblk3/1 -> cfblk4/1, cfblk5/2
  cfblk5/1 -> cfblk8/1
  cfblk6/1 -> cfblk11/1, cfblk5/1
  cfblk8/1 -> cfblk2/1

== system sampleModel1/cfblk114 ==
  cfblk1 : Inport
  cfblk12 : Inport  Port=2
  cfblk13 : Inport  Port=3
  Action Port : ActionPort  ActionPortLabel=if(u1 >= 0)
  cfblk10 : MinMax  Inputs=3
  cfblk11 : Subsystem
  cfblk16 : Delay
  cfblk17 : Delay
  cfblk3 : pid_lib/PID Controller (2DOF)  Controller=PID  Form=Parallel  TimeDomain=Discrete-time  UseExternalTs=off  SampleTime=-1  IntegratorMethod=Forward Euler  FilterMethod=Forward Euler  ControllerParametersSource=internal  P=1  I=1  D=0  UseFilter=on  N=100  b=1  c=1  TunerSelectOption=Transfer Function Based (PID Tuner App)  InitialConditionSource=internal  InitialConditionForIntegrator=0  InitialConditionForFilter=0  DifferentiatorICPrevScaledInput=0  ExternalReset=none  TrackingMode=off  Kt=1  LimitOutput=off  SatLimitsSource=internal  UpperSaturationLimit=inf  LowerSaturationLimit=-inf  LinearizeAsGain=off  AntiWindupMode=none  Kb=1  POutMin=[]  POutMax=[]  IOutMin=[]  IOutMax=[]  DOutMin=[]  DOutMax=[]  NOutMin=[]  NOutMax=[]  bOutMin=[]  bOutMax=[]  cOutMin=[]  cOutMax=[]  SumOutMin=[]  SumOutMax=[]  SaturationOutMin=[]  SaturationOutMax=[]  PParamMin=[]  PParamMax=[]  IParamMin=[]  IParamMax=[]  DParamMin=[]  DParamMax=[]  NParamMin=[]  NParamMax=[]  bParamMin=[]  bParamMax=[]  cParamMin=[]  cParamMax=[]  KbParamMin=[]  KbParamMax=[]  KtParamMin=[]  KtParamMax=[]  KbOutMin=[]  KbOutMax=[]  KtOutMin=[]  KtOutMax=[]  IntegratorOutMin=[]  IntegratorOutMax=[]  FilterOutMin=[]  FilterOutMax=[]  SumI1OutMin=[]  SumI1OutMax=[]  SumI2OutMin=[]  SumI2OutMax=[]  SumI3OutMin=[]  SumI3OutMax=[]  SumI4OutMin=[]  SumI4OutMax=[]  SumDOutMin=[]  SumDOutMax=[]  Sum1OutMin=[]  Sum1OutMax=[]  Sum2OutMin=[]  Sum2OutMax=[]  Sum3OutMin=[]  Sum3OutMax=[]  DifferentiatorOutMin=[]  DifferentiatorOutMax=[]  FilterDiffOutCoefMin=[]  FilterDiffOutCoefMax=[]  ReciprocalOutMin=[]  ReciprocalOutMax=[]  SumDenOutMin=[]  SumDenOutMax=[]  SumNumOutMin=[]  SumNumOutMax=[]  DivideOutMin=[]  DivideOutMax=[]  UdiffTsProdOutMin=[]  UdiffTsProdOutMax=[]  NTsProdOutMin=[]  NTsProdOutMax=[]  UintegralTsProdOutMin=[]  UintegralTsProdOutMax=[]  UngainTsProdOutMin=[]  UngainTsProdOutMax=[]  IntegratorContinuousStateAttributes=''  IntegratorStateMustResolveToSignalObject=off  IntegratorRTWStateStorageClass=Auto  FilterContinuousStateAttributes=''  FilterStateMustResolveToSignalObject=off  FilterRTWStateStorageClass=Auto  ParallelPVariant=InternalParameters  IdealPVariant=Disabled  IVariant=InternalParameters  DVariant=InternalParameters  bVariant=InternalParameters  cVariant=InternalParameters  IntegratorVariant=Discrete  SatVariant=Disabled  AWVariant=Passthrough  PCopyVariant=Disabled  TRVariant=Disabled  FdbkBlocksVariant=Forward  IdealPFdbkVariant=Disabled  SatFdbkVariant=Disabled  DerivativeFilterVariant=ForwardEulerFilter  NVariant=InternalParameters  NCopyVariant=Disabled  FilterICVariant=InternalICsFilter  IntegratorICVariant=InternalICs  ExternalResetVariant=Disabled  TRSumVariant=Passthrough  SumFdbkVariant=Disabled  SumVariant=Sum_PID  TsampFilterVariant=InternalTs  TsampNgainVariant=Passthrough  TsampIntegralVariant=Passthrough  ExternalSaturationOutDataTypeStr=Inherit: Same as second input
      settings: SourceProductBaseCode=SL
  cfblk4 : DotProduct  InputSameDT=on  OutDataTypeStr=Inherit: Inherit via internal rule
  cfblk5 : Squeeze
  cfblk6 : Math  Operator=log  SaturateOnIntegerOverflow=on
  cfblk7 : Product
  cfblk8 : Sin  TimeSource=Use external signal  SampleTime=0
  cfblk9 : Squeeze
  cfblk2 : Outport
  cfblk14 : Outport  Port=2
  cfblk15 : Outport  Port=3
  wires:
  cfblk6/1 -> cfblk4/1, cfblk8/1
  cfblk11/1(cfblk2) -> cfblk15/1
  cfblk12/1 -> cfblk9/1
  cfblk10/1 -> cfblk6/1
  cfblk11/2(cfblk15) -> cfblk7/1
  cfblk11/3(cfblk16) -> cfblk5/1
  cfblk13/1 -> cfblk2/1
  cfblk1/1 -> cfblk11/3(cfblk14), cfblk4/2
  cfblk7/1 -> cfblk3/1, cfblk17/1
  cfblk4/1 -> cfblk14/1
  cfblk3/1 -> cfblk10/1
  cfblk5/1 -> cfblk10/2
  cfblk11/4(cfblk17) -> cfblk3/2, cfblk7/2
  cfblk9/1 -> cfblk10/3
  cfblk8/1 -> cfblk16/1
  cfblk16/1 -> cfblk11/1(cfblk1)
  cfblk17/1 -> cfblk11/2(cfblk13)

== system sampleModel1/cfblk115 ==
  cfblk1 : Inport
  Action Port : ActionPort  ActionPortLabel=else
  cfblk10 : Constant  Value=[-120845132.391435]  SampleTime=1
  cfblk11 : Constant  Value=[980622646.799436]  SampleTime=1
  cfblk12 : Subsystem
  cfblk13 : If  IfExpression=u1 >= 0  SampleTime=1
  cfblk14 : Subsystem  TreatAsAtomicUnit=on
  cfblk15 : Subsystem  TreatAsAtomicUnit=on
  cfblk16 : Delay
  cfblk17 : Delay
  cfblk3 : DiscreteStateSpace  SampleTime=-1
  cfblk4 : Sin  TimeSource=Use external signal  SampleTime=0
  cfblk5 : Reshape
  cfblk6 : Sum  Inputs=+
  cfblk7 : Product  Inputs=**
  cfblk8 : Constant  Value=[404818103.909219]  SampleTime=1
  cfblk9 : Constant  Value=[422022460.064357]  SampleTime=1
  cfblk2 : Outport
  wires:
  cfblk6/1 -> cfblk2/1
  cfblk8/1 -> cfblk14/1(cfblk1)
  cfblk15/1(cfblk2) -> cfblk14/2(cfblk11)
  cfblk3/1 -> cfblk5/1
  cfblk5/1 -> cfblk7/1
  cfblk7/1 -> cfblk15/1(cfblk1)
  cfblk11/1 -> cfblk13/1
  cfblk1/1 -> cfblk3/1, cfblk15/2(cfblk9)
  cfblk9/1 -> cfblk7/2
  cfblk10/1 -> cfblk12/2(cfblk9)
  cfblk14/1(cfblk2) -> cfblk12/3(cfblk10)
  cfblk12/1(cfblk2) -> cfblk4/1
  cfblk14/2(cfblk12) -> cfblk6/1, cfblk17/1
  cfblk13/1 -> cfblk14/Action
  cfblk13/2 -> cfblk15/Action
  cfblk4/1 -> cfblk16/1
  cfblk16/1 -> cfblk12/1(cfblk1)
  cfblk17/1 -> cfblk15/3(cfblk10)

== system sampleModel1/cfblk73 ==
  cfblk1 : Inport
  cfblk10 : Constant  Value=[-82302343.640138]  SampleTime=1
  cfblk11 : Constant  Value=[93611437.477936]  SampleTime=1
  cfblk12 : Constant  Value=[-536811226.582952]  SampleTime=1
  cfblk13 : Constant  Value=[248120176.347379]  SampleTime=1
  cfblk14 : Constant  Value=[-208969568.662814]  SampleTime=1
  cfblk15 : If  IfExpression=u1 >= 0  SampleTime=1
  cfblk17 : Subsystem  TreatAsAtomicUnit=on
  cfblk18 : Subsystem  TreatAsAtomicUnit=on
  cfblk19 : Delay  SampleTime=1
  cfblk3 : Product
  cfblk4 : Assignment  DiagnosticForDimensions=Warning  IndexOptions=Index vector (dialog)  Indices=1  OutputSizes=1
  cfblk5 : Polyval  Coefs=[ +2.081618890e-019, -1.441693666e-014, +4.719686976e-010, -8.536869453e-006, +1.621573104e-001, -8.087801117e+001 ]
  cfblk6 : Sqrt  SaturateOnIntegerOverflow=on
  cfblk7 : Sum  Inputs=-+
  cfblk8 : Trigonometry
  cfblk9 : Sin  TimeSource=Use external signal  SampleTime=0
  cfblk2 : Outport
  cfblk16 : Outport  Port=2
  wires:
  cfblk11/1 -> cfblk4/1
  cfblk3/1 -> cfblk5/1
  cfblk17/1(cfblk2) -> cfblk4/2
  cfblk6/1 -> cfblk2/1
  cfblk9/1 -> cfblk3/1
  cfblk1/1 -> cfblk7/1
  cfblk10/1 -> cfblk8/1
  cfblk18/1(cfblk2) -> cfblk6/1
  cfblk7/1 -> cfblk9/1
  cfblk8/1 -> cfblk7/2
  cfblk13/1 -> cfblk15/1
  cfblk12/1 -> cfblk18/1(cfblk1), cfblk17/3(cfblk6)
  cfblk4/1 -> cfblk16/1
  cfblk14/1 -> cfblk18/2(cfblk9)
  cfblk5/1 -> cfblk17/1(cfblk1)
  cfblk18/2(cfblk10) -> cfblk17/2(cfblk5)
  cfblk15/1 -> cfblk17/Action
  cfblk15/2 -> cfblk18/Action
  cfblk17/2(cfblk7) -> cfblk19/1
  cfblk19/1 -> cfblk3/2

== system sampleModel1/cfblk88 ==
  cfblk1 : Inport
  cfblk8 : Inport  Port=2
  cfblk9 : Inport  Port=3
  cfblk10 : Inport  Port=4
  Action Port : ActionPort  ActionPortLabel=if(u1 >= 0)
  cfblk3 : Sin  TimeSource=Use external signal  SampleTime=0
  cfblk4 : Sum
  cfblk5 : Constant  Value=[596701728.227905]  SampleTime=1
  cfblk6 : Constant  Value=[367431144.816716]  SampleTime=1
  cfblk7 : Constant  Value=[445449079.313532]  SampleTime=1
  cfblk2 : Outport
  wires:
  cfblk7/1 -> cfblk2/1
  cfblk8/1 -> cfblk3/1
  cfblk6/1 -> cfblk4/1
  cfblk3/1 -> cfblk4/2

== system sampleModel1/cfblk89 ==
  cfblk1 : Inport
  cfblk12 : Inport  Port=2
  cfblk13 : Inport  Port=3
  cfblk14 : Inport  Port=4
  Action Port : ActionPort  ActionPortLabel=else
  cfblk10 : Constant  Value=[-411867332.482743]  SampleTime=1
  cfblk11 : Subsystem
  cfblk16 : Delay
  cfblk3 : Assignment  DiagnosticForDimensions=Warning  IndexOptions=Index vector (dialog)  Indices=1  OutputSizes=1
  cfblk4 : Product  Inputs=*
  cfblk5 : DotProduct  InputSameDT=on  OutDataTypeStr=Inherit: Inherit via internal rule
  cfblk6 : Rounding
  cfblk7 : Polyval  Coefs=[ +2.081618890e-019, -1.441693666e-014, +4.719686976e-010, -8.536869453e-006, +1.621573104e-001, -8.087801117e+001 ]
  cfblk8 : ComplexToMagnitudeAngle
  cfblk9 : Sqrt  SaturateOnIntegerOverflow=on
  cfblk2 : Outport
  cfblk15 : Outport  Port=2
  wires:
  cfblk6/1 -> cfblk8/1
  cfblk1/1 -> cfblk7/1
  cfblk12/1 -> cfblk15/1
  cfblk13/1 -> cfblk9/1
  cfblk9/1 -> cfblk4/1
  cfblk8/1 -> cfblk5/1
  cfblk5/1 -> cfblk3/1
  cfblk4/1 -> cfblk5/2
  cfblk14/1 -> cfblk11/1(cfblk1)
  cfblk8/2 -> cfblk2/1
  cfblk3/1 -> cfblk11/2(cfblk11)
  cfblk7/1 -> cfblk6/1
  cfblk11/1(cfblk2) -> cfblk16/1
  cfblk16/1 -> cfblk3/2

== system sampleModel1/cfblk90 ==
  cfblk1 : Inport
  cfblk11 : Inport  Port=2
  cfblk12 : Inport  Port=3
  Action Port : ActionPort  ActionPortLabel=if(u1 >= 0)
  cfblk10 : Constant  Value=[-176812973.184931]  SampleTime=1
  cfblk3 : pid_lib/PID Controller  Controller=PID  Form=Parallel  TimeDomain=Discrete-time  UseExternalTs=off  SampleTime=-1  IntegratorMethod=Forward Euler  FilterMethod=Forward Euler  ControllerParametersSource=internal  P=1  I=1  D=0  UseFilter=on  N=100  TunerSelectOption=Transfer Function Based (PID Tuner App)  InitialConditionSource=internal  InitialConditionForIntegrator=0  InitialConditionForFilter=0  DifferentiatorICPrevScaledInput=0  ExternalReset=none  TrackingMode=off  Kt=1  LimitOutput=off  SatLimitsSource=internal  UpperSaturationLimit=inf  LowerSaturationLimit=-inf  LinearizeAsGain=off  AntiWindupMode=none  Kb=1  POutMin=[]  POutMax=[]  IOutMin=[]  IOutMax=[]  DOutMin=[]  DOutMax=[]  NOutMin=[]  NOutMax=[]  SumOutMin=[]  SumOutMax=[]  SaturationOutMin=[]  SaturationOutMax=[]  PParamMin=[]  PParamMax=[]  IParamMin=[]  IParamMax=[]  DParamMin=[]  DParamMax=[]  NParamMin=[]  NParamMax=[]  KbParamMin=[]  KbParamMax=[]  KtParamMin=[]  KtParamMax=[]  KbOutMin=[]  KbOutMax=[]  KtOutMin=[]  KtOutMax=[]  IntegratorOutMin=[]  IntegratorOutMax=[]  FilterOutMin=[]  FilterOutMax=[]  SumI1OutMin=[]  SumI1OutMax=[]  SumI2OutMin=[]  SumI2OutMax=[]  SumI3OutMin=[]  SumI3OutMax=[]  SumI4OutMin=[]  SumI4OutMax=[]  SumDOutMin=[]  SumDOutMax=[]  DifferentiatorOutMin=[]  DifferentiatorOutMax=[]  FilterDiffOutCoefMin=[]  FilterDiffOutCoefMax=[]  ReciprocalOutMin=[]  ReciprocalOutMax=[]  SumDenOutMin=[]  SumDenOutMax=[]  SumNumOutMin=[]  SumNumOutMax=[]  DivideOutMin=[]  DivideOutMax=[]  UdiffTsProdOutMin=[]  UdiffTsProdOutMax=[]  NTsProdOutMin=[]  NTsProdOutMax=[]  UintegralTsProdOutMin=[]  UintegralTsProdOutMax=[]  UngainTsProdOutMin=[]  UngainTsProdOutMax=[]  IntegratorContinuousStateAttributes=''  IntegratorStateMustResolveToSignalObject=off  IntegratorRTWStateStorageClass=Auto  FilterContinuousStateAttributes=''  FilterStateMustResolveToSignalObject=off  FilterRTWStateStorageClass=Auto  ParallelPVariant=InternalParameters  IdealPVariant=Disabled  IVariant=InternalParameters  DVariant=InternalParameters  IntegratorVariant=Discrete  SatVariant=Disabled  AWVariant=Passthrough  PCopyVariant=Disabled  TRVariant=Disabled  FdbkBlocksVariant=Forward  IdealPFdbkVariant=Disabled  SatFdbkVariant=Disabled  DerivativeFilterVariant=ForwardEulerFilter  NVariant=InternalParameters  NCopyVariant=Disabled  FilterICVariant=InternalICsFilter  IntegratorICVariant=InternalICs  ExternalResetVariant=Disabled  TRSumVariant=Passthrough  SumFdbkVariant=Disabled  SumVariant=Sum_PID  TsampFilterVariant=InternalTs  TsampNgainVariant=Passthrough  TsampIntegralVariant=Passthrough  ExternalSaturationOutDataTypeStr=Inherit: Same as second input
  cfblk4 : MinMax  Inputs=2
  cfblk5 : simulink/Math Operations/Slider Gain  gain=1  low=0  high=2
  cfblk6 : UnaryMinus
  cfblk7 : Signum
  cfblk8 : Constant  Value=[-511669426.419441]  SampleTime=1
  cfblk9 : Constant  Value=[360356742.461004]  SampleTime=1
  cfblk2 : Outport
  cfblk13 : Outport  Port=2
  cfblk14 : Outport  Port=3
  wires:
  cfblk8/1 -> cfblk13/1
  cfblk9/1 -> cfblk5/1
  cfblk1/1 -> cfblk6/1
  cfblk12/1 -> cfblk7/1
  cfblk11/1 -> cfblk3/1
  cfblk10/1 -> cfblk4/1
  cfblk5/1 -> cfblk4/2
  cfblk3/1 -> cfblk2/1
  cfblk7/1 -> cfblk14/1

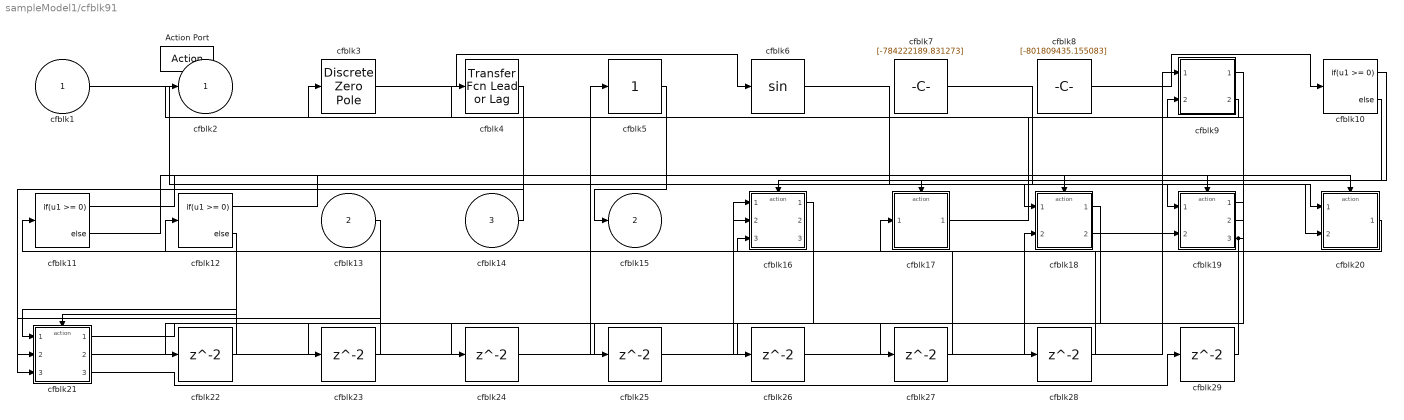
== system sampleModel1/cfblk91 ==
  cfblk1 : Inport
  cfblk13 : Inport  Port=2
  cfblk14 : Inport  Port=3
  Action Port : ActionPort  ActionPortLabel=else
  cfblk10 : If  IfExpression=u1 >= 0  SampleTime=1
  cfblk11 : If  IfExpression=u1 >= 0  SampleTime=1
  cfblk12 : If  IfExpression=u1 >= 0  SampleTime=1
  cfblk16 : Subsystem  TreatAsAtomicUnit=on
  cfblk17 : Subsystem  TreatAsAtomicUnit=on
  cfblk18 : Subsystem  TreatAsAtomicUnit=on
  cfblk19 : Subsystem  TreatAsAtomicUnit=on
  cfblk20 : Subsystem  TreatAsAtomicUnit=on
  cfblk21 : Subsystem  TreatAsAtomicUnit=on
  cfblk{22..29} (8 alike) : Delay
  cfblk3 : DiscreteZeroPole  Poles=[0 0.5]  Gain=1  SampleTime=-1
  cfblk4 : simulink/Discrete/Transfer Fcn Lead or Lag  PoleZ=0.95  ZeroZ=0.75  ICPrevOutput=0.0  ICPrevInput=0.0  DoSatur=off
      settings: SourceProductBaseCode=SL
  cfblk5 : simulink/Math Operations/Slider Gain  gain=1  low=0  high=2
  cfblk6 : Trigonometry
  cfblk7 : Constant  Value=[-784222189.831273]  SampleTime=1
  cfblk8 : Constant  Value=[-801809435.155083]  SampleTime=1
  cfblk9 : Subsystem
  cfblk2 : Outport
  cfblk15 : Outport  Port=2
  wires:
  cfblk1/1 -> cfblk20/1(cfblk1)
  cfblk5/1 -> cfblk15/1
  cfblk6/1 -> cfblk19/1(cfblk1)
  cfblk3/1 -> cfblk6/1
  cfblk14/1 -> cfblk4/1
  cfblk8/1 -> cfblk10/1
  cfblk13/1 -> cfblk21/2(cfblk10)
  cfblk4/1 -> cfblk21/3(cfblk11)
  cfblk20/1(cfblk2) -> cfblk17/1(cfblk1)
  cfblk21/2(cfblk12) -> cfblk5/1
  cfblk18/2(cfblk13) -> cfblk19/2(cfblk6)
  cfblk17/1(cfblk2) -> cfblk9/2(cfblk8)
  cfblk9/1(cfblk2) -> cfblk18/1(cfblk1)
  cfblk19/3(cfblk8) -> cfblk2/1, cfblk27/1, cfblk28/1
  cfblk7/1 -> cfblk20/2(cfblk11)
  cfblk9/2(cfblk9) -> cfblk3/1
  cfblk10/1 -> cfblk16/Action
  cfblk10/2 -> cfblk17/Action
  cfblk11/1 -> cfblk18/Action
  cfblk11/2 -> cfblk19/Action
  cfblk12/1 -> cfblk20/Action
  cfblk12/2 -> cfblk21/Action
  cfblk18/1(cfblk2) -> cfblk22/1
  cfblk22/1 -> cfblk21/1(cfblk1)
  cfblk21/1(cfblk2) -> cfblk23/1
  cfblk23/1 -> cfblk11/1
  cfblk19/1(cfblk2) -> cfblk24/1
  cfblk24/1 -> cfblk16/1(cfblk1)
  cfblk16/1(cfblk2) -> cfblk25/1
  cfblk25/1 -> cfblk9/1(cfblk1)
  cfblk19/2(cfblk7) -> cfblk26/1
  cfblk26/1 -> cfblk18/2(cfblk12)
  cfblk27/1 -> cfblk16/2(cfblk12)
  cfblk28/1 -> cfblk16/3(cfblk13)
  cfblk21/3(cfblk13) -> cfblk29/1
  cfblk29/1 -> cfblk12/1

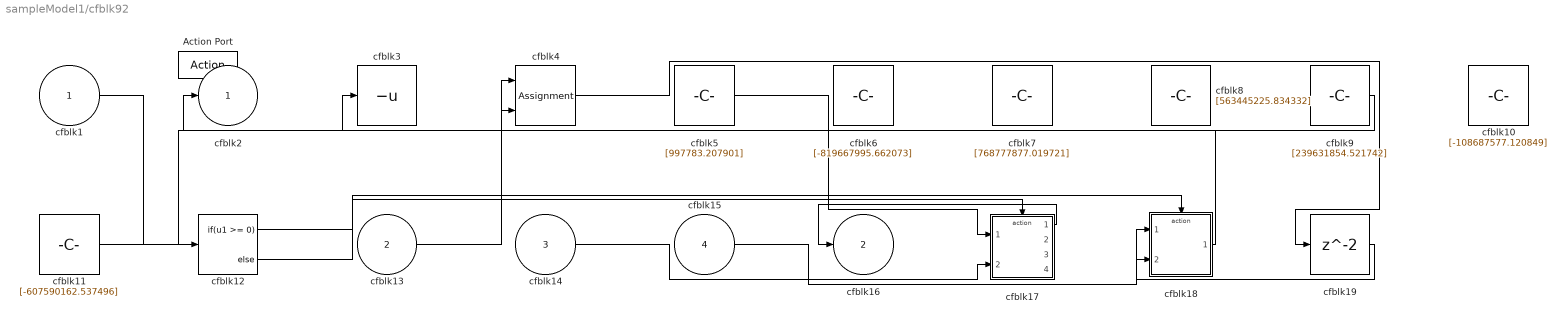
== system sampleModel1/cfblk92 ==
  cfblk1 : Inport
  cfblk13 : Inport  Port=2
  cfblk14 : Inport  Port=3
  cfblk15 : Inport  Port=4
  Action Port : ActionPort  ActionPortLabel=if(u1 >= 0)
  cfblk10 : Constant  Value=[-108687577.120849]  SampleTime=1
  cfblk11 : Constant  Value=[-607590162.537496]  SampleTime=1
  cfblk12 : If  IfExpression=u1 >= 0  SampleTime=1
  cfblk17 : Subsystem  TreatAsAtomicUnit=on
  cfblk18 : Subsystem  TreatAsAtomicUnit=on
  cfblk19 : Delay
  cfblk3 : UnaryMinus
  cfblk4 : Assignment  DiagnosticForDimensions=Warning  IndexOptions=Index vector (dialog)  Indices=1  OutputSizes=1
  cfblk5 : Constant  Value=[997783.207901]  SampleTime=1
  cfblk6 : Constant  Value=[-819667995.662073]  SampleTime=1
  cfblk7 : Constant  Value=[768777877.019721]  SampleTime=1
  cfblk8 : Constant  Value=[563445225.834332]  SampleTime=1
  cfblk9 : Constant  Value=[239631854.521742]  SampleTime=1
  cfblk2 : Outport
  cfblk16 : Outport  Port=2
  wires:
  cfblk1/1 -> cfblk12/1
  cfblk17/1(cfblk2) -> cfblk16/1
  cfblk9/1 -> cfblk2/1
  cfblk18/1(cfblk2) -> cfblk4/1
  cfblk5/1 -> cfblk17/1(cfblk1)
  cfblk11/1 -> cfblk3/1
  cfblk15/1 -> cfblk18/1(cfblk1)
  cfblk14/1 -> cfblk17/2(cfblk7)
  cfblk13/1 -> cfblk4/2
  cfblk12/1 -> cfblk17/Action
  cfblk12/2 -> cfblk18/Action
  cfblk4/1 -> cfblk19/1
  cfblk19/1 -> cfblk18/2(cfblk8)

== system sampleModel1/cfblk93 ==
  cfblk1 : Inport
  cfblk14 : Inport  Port=2
  cfblk15 : Inport  Port=3
  cfblk16 : Inport  Port=4
  Action Port : ActionPort  ActionPortLabel=else
  cfblk10 : Constant  Value=[-520245053.016234]  SampleTime=1
  cfblk11 : Constant  Value=[-41191192.796015]  SampleTime=1
  cfblk12 : Constant  Value=[869418475.827621]  SampleTime=1
  cfblk13 : Constant  Value=[417817957.803642]  SampleTime=1
  cfblk3 : PermuteDimensions
  cfblk4 : Sqrt  SaturateOnIntegerOverflow=on
  cfblk5 : Math  SaturateOnIntegerOverflow=on
  cfblk6 : MinMax  Inputs=2
  cfblk7 : Product
  cfblk8 : Sum  Inputs=+
  cfblk9 : Constant  Value=[729345092.766074]  SampleTime=1
  cfblk2 : Outport
  wires:
  cfblk1/1 -> cfblk8/1
  cfblk3/1 -> cfblk4/1
  cfblk11/1 -> cfblk7/1
  cfblk6/1 -> cfblk3/1
  cfblk8/1 -> cfblk6/1
  cfblk4/1 -> cfblk2/1
  cfblk12/1 -> cfblk5/1
  cfblk10/1 -> cfblk6/2
  cfblk13/1 -> cfblk7/2

== system sampleModel1/cfblk94 ==
  cfblk1 : Inport
  cfblk8 : Inport  Port=2
  Action Port : ActionPort  ActionPortLabel=if(u1 >= 0)
  cfblk3 : simulink/Discrete/Tapped Delay  vinit=0.0  samptime=-1  NumDelays=1  DelayOrder=Oldest  includeCurrent=off
  cfblk4 : PermuteDimensions
  cfblk5 : Signum
  cfblk6 : Reshape
  cfblk7 : Constant  Value=[324703479.256078]  SampleTime=1
  cfblk2 : Outport
  wires:
  cfblk1/1 -> cfblk4/1
  cfblk7/1 -> cfblk2/1
  cfblk6/1 -> cfblk3/1
  cfblk5/1 -> cfblk6/1
  cfblk4/1 -> cfblk5/1

== system sampleModel1/cfblk95 ==
  cfblk1 : Inport
  cfblk9 : Inport  Port=2
  cfblk10 : Inport  Port=3
  Action Port : ActionPort  ActionPortLabel=else
  cfblk13 : Delay
  cfblk14 : Delay
  cfblk3 : Sqrt  Operator=rSqrt  AlgorithmType=Newton-Raphson  SaturateOnIntegerOverflow=on
  cfblk4 : MinMax  Function=max  Inputs=3
  cfblk5 : Product
  cfblk6 : Constant  Value=[-396093061.745536]  SampleTime=1
  cfblk7 : Constant  Value=[651930964.968488]  SampleTime=1
  cfblk8 : Subsystem
  cfblk2 : Outport
  cfblk11 : Outport  Port=2
  cfblk12 : Outport  Port=3
  wires:
  cfblk3/1 -> cfblk8/1(cfblk1)
  cfblk1/1 -> cfblk5/1, cfblk8/3(cfblk10)
  cfblk4/1 -> cfblk3/1
  cfblk9/1 -> cfblk2/1, cfblk8/2(cfblk9)
  cfblk5/1 -> cfblk4/2
  cfblk10/1 -> cfblk12/1, cfblk8/4(cfblk11)
  cfblk7/1 -> cfblk4/3
  cfblk6/1 -> cfblk11/1
  cfblk8/1(cfblk2) -> cfblk13/1
  cfblk13/1 -> cfblk4/1
  cfblk8/2(cfblk12) -> cfblk14/1
  cfblk14/1 -> cfblk5/2

== system sampleModel1/cfblk96 ==
  cfblk1 : Inport
  cfblk12 : Inport  Port=2
  Action Port : ActionPort  ActionPortLabel=if(u1 >= 0)
  cfblk10 : Constant  Value=[174806800.248188]  SampleTime=1
  cfblk11 : Subsystem
  cfblk15 : Delay
  cfblk3 : Squeeze
  cfblk4 : Assignment  DiagnosticForDimensions=Warning  IndexOptions=Index vector (dialog)  Indices=1  OutputSizes=1
  cfblk5 : Product  Inputs=*
  cfblk6 : Sqrt  SaturateOnIntegerOverflow=on
  cfblk7 : Sin  TimeSource=Use external signal  SampleTime=0
  cfblk8 : Constant  Value=[-716674039.395082]  SampleTime=1
  cfblk9 : Constant  Value=[-299239255.173062]  SampleTime=1
  cfblk2 : Outport
  cfblk13 : Outport  Port=2
  cfblk14 : Outport  Port=3
  wires:
  cfblk8/1 -> cfblk14/1
  cfblk12/1 -> cfblk11/1(cfblk1)
  cfblk3/1 -> cfblk13/1
  cfblk6/1 -> cfblk2/1
  cfblk7/1 -> cfblk3/1
  cfblk9/1 -> cfblk5/1
  cfblk10/1 -> cfblk11/3(cfblk13)
  cfblk5/1 -> cfblk6/1
  cfblk1/1 -> cfblk11/4(cfblk14)
  cfblk11/1(cfblk2) -> cfblk7/1
  cfblk11/2(cfblk15) -> cfblk4/1
  cfblk11/3(cfblk16) -> cfblk4/2
  cfblk4/1 -> cfblk15/1
  cfblk15/1 -> cfblk11/2(cfblk12)

== system sampleModel1/cfblk97 ==
  cfblk1 : Inport
  cfblk10 : Inport  Port=2
  Action Port : ActionPort  ActionPortLabel=else
  cfblk3 : Math  Operator=mod  SaturateOnIntegerOverflow=on
  cfblk4 : Squeeze
  cfblk5 : Product  Inputs=*
  cfblk6 : Product
  cfblk7 : Constant  Value=[-759474458.440043]  SampleTime=1
  cfblk8 : Constant  Value=[-306702628.898907]  SampleTime=1
  cfblk9 : Constant  Value=[149233126.761950]  SampleTime=1
  cfblk2 : Outport
  cfblk11 : Outport  Port=2
  wires:
  cfblk8/1 -> cfblk3/1
  cfblk3/1 -> cfblk11/1
  cfblk6/1 -> cfblk3/2
  cfblk7/1 -> cfblk6/1
  cfblk9/1 -> cfblk4/1
  cfblk4/1 -> cfblk5/1
  cfblk10/1 -> cfblk2/1
  cfblk1/1 -> cfblk6/2

== system sampleModel1/cfblk98 ==
  cfblk1 : Inport
  cfblk7 : Inport  Port=2
  Action Port : ActionPort  ActionPortLabel=if(u1 >= 0)
  cfblk3 : Sum  Inputs=-+
  cfblk4 : ComplexToMagnitudeAngle
  cfblk5 : simulink/Math Operations/Slider Gain  gain=1  low=0  high=2
  cfblk6 : Constant  Value=[-340440663.432103]  SampleTime=1
  cfblk2 : Outport
  wires:
  cfblk1/1 -> cfblk5/1
  cfblk3/1 -> cfblk4/1
  cfblk6/1 -> cfblk2/1
  cfblk5/1 -> cfblk3/1
  cfblk7/1 -> cfblk3/2
